simulink model "test_haptic_skin_scheduler_vtrial_m8_forfigure"  (R2023a)
settings: Solver=FixedStepAuto  StartTime=1.0  StopTime=2.0  FixedStep=0.0001  RelTol=1e-3
model workspace (MAT data in the model file):
  amp1 = 80
settings Model: Creator=Daneel  LastModifiedBy=HP

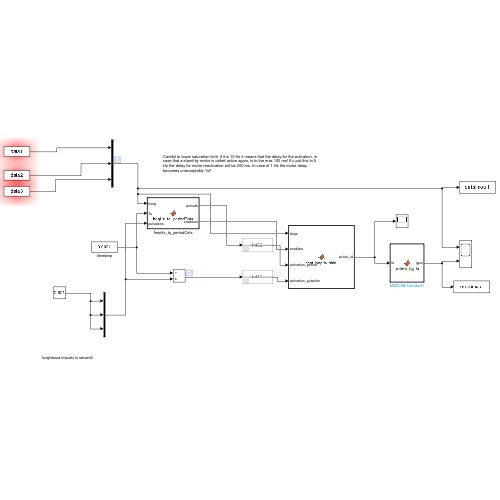
[thumbnail: Simulink's stored preview of the top-level diagram]
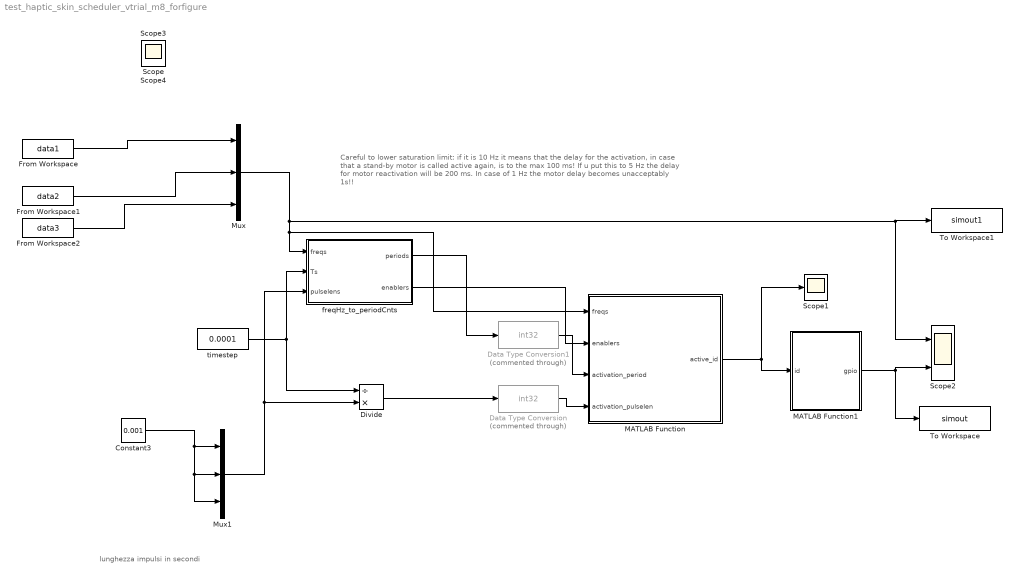
== system test_haptic_skin_scheduler_vtrial_m8_forfigure ==
  note: Careful to lower saturation limit: if it is 10 Hz it means that the delay for the activation, in case that a stand-by motor is called active again, is to the max 100 ms! If u put this to 5 Hz the delay for motor reactivation will be 200 ms. In case of 1 Hz the motor delay becomes unacceptably 1s!!
  note: lunghezza impulsi in secondi
  Constant3 : Constant  Value=0.001
  Data Type Conversion : DataTypeConversion  Commented=through  OutDataTypeStr=int32  SaturateOnIntegerOverflow=off  RndMeth=Floor
  Data Type Conversion1 : DataTypeConversion  Commented=through  OutDataTypeStr=int32  SaturateOnIntegerOverflow=off  RndMeth=Floor
  Divide : Product  Inputs=/*
  From Workspace : FromWorkspace  VariableName=data1  SampleTime=-1
  From Workspace1 : FromWorkspace  VariableName=data2  SampleTime=-1
  From Workspace2 : FromWorkspace  VariableName=data3  SampleTime=-1
  MATLAB Function : MATLAB Function  TreatAsAtomicUnit=on
  MATLAB Function1 : MATLAB Function  TreatAsAtomicUnit=on
  Mux : Mux  Inputs=3
  Mux1 : Mux  Inputs=3
  Scope{,1,3..4} (4 alike) : Scope
  Scope2 : Scope  NumInputPorts=2
  To Workspace : ToWorkspace  VariableName=simout  SampleTime=-1
      settings: Save2DSignal=2-D array (concatenate along first dimension)
  To Workspace1 : ToWorkspace  VariableName=simout1  SampleTime=-1
      settings: Save2DSignal=2-D array (concatenate along first dimension)
  freqHz_to_periodCnts : MATLAB Function  TreatAsAtomicUnit=on
  timestep : Constant  Value=0.0001
  wires:
  Mux1/1 -> freqHz_to_periodCnts/3(pulselens), Divide/2
  MATLAB Function/1(active_id) -> MATLAB Function1/1(id), Scope1/1
  timestep/1 -> Divide/1, freqHz_to_periodCnts/2(Ts)
  Mux/1 -> MATLAB Function/1(freqs), freqHz_to_periodCnts/1(freqs), To Workspace1/1, Scope2/1
  Data Type Conversion/1 -> MATLAB Function/4(activation_pulselen)
  Data Type Conversion1/1 -> MATLAB Function/3(activation_period)
  freqHz_to_periodCnts/1(periods) -> Data Type Conversion1/1
  Divide/1 -> Data Type Conversion/1
  MATLAB Function1/1(gpio) -> To Workspace/1, Scope2/2
  Constant3/1 -> Mux1/3, Mux1/2, Mux1/1
  freqHz_to_periodCnts/2(enablers) -> MATLAB Function/2(enablers)
  From Workspace/1 -> Mux/1
  From Workspace1/1 -> Mux/2
  From Workspace2/1 -> Mux/3

== matlab function test_haptic_skin_scheduler_vtrial_m8_forfigure/MATLAB Function1 ==
  data: id input; gpio output
function gpio = activeid2gpio(id)

gpio = zeros(1,3);
if(id>0)
    gpio(id)=1;
end

== matlab function test_haptic_skin_scheduler_vtrial_m8_forfigure/MATLAB Function ==
  data: freqs input; enablers input; activation_period input; active_id output; activation_pulselen input
function active_id  = test_haptic_skin(freqs,enablers,activation_period, activation_pulselen)

%activation_period e activation_pulse len sono vettori
%active_id è un segnale scalare di uscita: 0 nessun motore attivo,
%altrimenti id del motore attivo

persistent pulse_on_cnt;
persistent pulse_on_id;
persistent activation_cnt;

if(isempty(activation_cnt))
    activation_cnt = zeros(1,length(activation_period));
    pulse_on_cnt = 0;
    pulse_on_id = 0;
end

N = length(activation_period);
active_id = 0;

min = 0;
min_id = 0;

%try this new: this is the real strategy that was proposed!

for i=1:N
    %decrease counters
    activation_cnt(i)=enablers(i)*(activation_cnt(i)-1*enablers(i));

    %find the most waiting motor
    if(activation_cnt(i)<min)
        min = activation_cnt(i)/activation_period(i);
        min_id = i;
    end
end

%activate the motor
if(pulse_on_cnt == 0) % se nessun impulso attivo
    if(min<0) %almeno un motore in lista per attivazione impulso
        pulse_on_id = min_id; %imposto nuovo impulso
        pulse_on_cnt = activation_pulselen(pulse_on_id);
    else
        pulse_on_id = 0;
    end
else % se impulso attivo
    pulse_on_cnt = pulse_on_cnt-1;
    if(pulse_on_cnt==0) %se evento fine impulso
         activation_cnt(pulse_on_id) = activation_period(pulse_on_id); %reimposto counter del motore che ha appena terminato l'impulso
    end
end

active_id=pulse_on_id;

%check if it is under saturation
% if active_id~=0
%     active_id=active_id*(enablers(active_id));
% end

== matlab function test_haptic_skin_scheduler_vtrial_m8_forfigure/freqHz_to_periodCnts ==
  data: freqs input; periods output; Ts input; pulselens input; enablers output
function [periods,enablers]   = freqHz_to_periodCnts(freqs, Ts, pulselens) %frequenze in Hz, timestep in secondi
fthresh=10;
N = length(freqs);
periods = zeros(1,N);
    for i=1:N
          if(freqs(i)<fthresh)
              freqs(i) = fthresh; %saturazione per evitare div zero e periodo infinito
          end
          periods(i) = 1/(freqs(i)*Ts)-pulselens(i)/Ts;
    end
enablers=(freqs>fthresh);
end
